simulink model "labFiveSimu"  (R2016a)
settings: Solver=VariableStepAuto  StartTime=0.0  StopTime=10.0  RelTol=1e-3
libraries: simulink x1
settings Model: Creator=farnamadelkhani  LastModifiedBy=farnamadelkhani

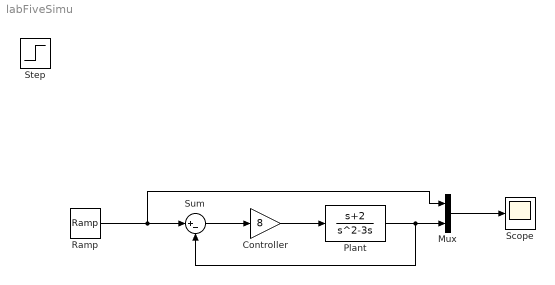
== system labFiveSimu ==
  Controller : Gain  Gain=8
  Mux : Mux  Inputs=2
  Plant : TransferFcn  Numerator=[1 2]  Denominator=[1 -3 0]
  Ramp : simulink/Sources/Ramp  slope=1  start=0  X0=0
  Scope : Scope
  Step : Step  SampleTime=0
  Sum : Sum  Inputs=|+-
  wires:
  Sum/1 -> Controller/1
  Controller/1 -> Plant/1
  Plant/1 -> Mux/2, Sum/2
  Mux/1 -> Scope/1
  Ramp/1 -> Mux/1, Sum/1
